simulink model "fwv_2020bn"  (R2020b)
settings: Solver=daessc  StartTime=0.0  StopTime=12  FixedStep=0.01  MaxStep=0.01  RelTol=1e-3  AbsTol=1e-3  EnableMultiTasking=on
model workspace: external: MATLAB File main.m (data not in the file)
values from neighbouring files (symbols this model uses):
  A_D = 1.5    [main.m]    (also in param.m; params.m)
  A_L = 1.8    [main.m]    (also in param.m; params.m)
  c_bar = S/R    (= 0.0357142857143)    [main.m]    (also in param.m = 0.0251327412287; params.m)
  C_D0 = 0.45    [main.m]    (also in param.m; params.m)
  m = 2    [rbf_pid.m]
  r00 = double(int(f,[0,1]))    [main.m]    (also in param.m = 1; params.m = 0.933333333333)
  r11 = double(int(x*f,[0,1]))    [main.m]    (also in param.m = double(int(curv(x)*(x+1/9),0,1)); params.m = 0.481185185185)
  r22 = double(int(x^2*f,[0,1]))    [main.m]    (also in param.m = double(int(curv(x)*(x+1/9)^2,0,1)); params.m = 0.304750617284)
  r33 = double(int(x^3*f,[0,1]))    [main.m]    (also in param.m = double(int(curv(x)*(x+1/9)^3,0,1)); params.m = 0.218568691358)
  r_cp = Rw*r33/r22    [main.m]    (also in param.m; params.m = 0.10758076225)
  rho = 1.205    [main.m]    (also in param.m; params.m)
  Rw = 0.15    [main.m]    (also in param.m = 0.075; params.m)
  z00 = double(int(f^2,[0,1]))    [main.m]    (also in param.m = double(int(curv(x)^2,0,1)); params.m = 1.00177777778)
  z11 = double(int(x*f^2,[0,1]))    [main.m]    (also in param.m = double(int(curv(x)^2*(x+1/9),0,1)); params.m = 0.484918518519)
  z22 = double(int(x^2*f^2,[0,1]))    [main.m]    (also in param.m = double(int(curv(x)^2*(x+1/9)^2,0,1)); params.m = 0.28785382716)
  zrd = double(int(f^4,[0,1]))    [main.m]    (also in param.m = double(int(curv(x)^4,0,1)); params.m = 1.29333866667)
undefined symbols (not defined in the file or in its folder): X, Y, Z
libraries: sm_lib x50, nesl_utility x45, pid_lib x5
(part 3 of 3)

== system fwv_2020bn/Controller/Subsystem/Outer PID ==
  In1 : Inport
  Demux : Demux  Outputs=3
  PID : Subsystem  mask{Kp=0.5, Ki=0.4, Kd=0.2, td=0}
  PID Controller1 : pid_lib/PID Controller  Controller=PID  Form=Parallel  TimeDomain=Continuous-time  UseExternalTs=off  SampleTime=-1  IntegratorMethod=Forward Euler  FilterMethod=Forward Euler  ControllerParametersSource=internal  P=0.3  I=0  D=0.3  UseFilter=on  N=25  TunerSelectOption=Transfer Function Based (PID Tuner App)  InitialConditionSource=internal  InitialConditionForIntegrator=0  InitialConditionForFilter=0  DifferentiatorICPrevScaledInput=0  ExternalReset=none  TrackingMode=off  Kt=1  LimitOutput=off  SatLimitsSource=internal  UpperSaturationLimit=inf  LowerSaturationLimit=-inf  LinearizeAsGain=on  AntiWindupMode=none  Kb=1  POutMin=[]  POutMax=[]  IOutMin=[]  IOutMax=[]  DOutMin=[]  DOutMax=[]  NOutMin=[]  NOutMax=[]  SumOutMin=[]  SumOutMax=[]  SaturationOutMin=[]  SaturationOutMax=[]  PParamMin=[]  PParamMax=[]  IParamMin=[]  IParamMax=[]  DParamMin=[]  DParamMax=[]  NParamMin=[]  NParamMax=[]  KbParamMin=[]  KbParamMax=[]  KtParamMin=[]  KtParamMax=[]  KbOutMin=[]  KbOutMax=[]  KtOutMin=[]  KtOutMax=[]  IntegratorOutMin=[]  IntegratorOutMax=[]  FilterOutMin=[]  FilterOutMax=[]  SumI1OutMin=[]  SumI1OutMax=[]  SumI2OutMin=[]  SumI2OutMax=[]  SumI3OutMin=[]  SumI3OutMax=[]  SumI4OutMin=[]  SumI4OutMax=[]  SumDOutMin=[]  SumDOutMax=[]  DifferentiatorOutMin=[]  DifferentiatorOutMax=[]  FilterDiffOutCoefMin=[]  FilterDiffOutCoefMax=[]  ReciprocalOutMin=[]  ReciprocalOutMax=[]  SumDenOutMin=[]  SumDenOutMax=[]  SumNumOutMin=[]  SumNumOutMax=[]  DivideOutMin=[]  DivideOutMax=[]  UdiffTsProdOutMin=[]  UdiffTsProdOutMax=[]  NTsProdOutMin=[]  NTsProdOutMax=[]  UintegralTsProdOutMin=[]  UintegralTsProdOutMax=[]  UngainTsProdOutMin=[]  UngainTsProdOutMax=[]  IntegratorContinuousStateAttributes=''  IntegratorStateMustResolveToSignalObject=off  IntegratorRTWStateStorageClass=Auto  FilterContinuousStateAttributes=''  FilterStateMustResolveToSignalObject=off  FilterRTWStateStorageClass=Auto  ParallelPVariant=InternalParameters  IdealPVariant=Disabled  IVariant=InternalParameters  DVariant=InternalParameters  IntegratorVariant=Continuous  SatVariant=Disabled  AWVariant=Passthrough  PCopyVariant=Disabled  TRVariant=Disabled  FdbkBlocksVariant=Forward  IdealPFdbkVariant=Disabled  SatFdbkVariant=Disabled  DerivativeFilterVariant=ContFilter  NVariant=InternalParameters  NCopyVariant=Disabled  FilterICVariant=InternalICsFilter  IntegratorICVariant=InternalICs  ExternalResetVariant=Disabled  TRSumVariant=Passthrough  SumFdbkVariant=Disabled  SumVariant=Sum_PID  TsampFilterVariant=InternalTs  TsampNgainVariant=Passthrough  TsampIntegralVariant=Passthrough  ExternalSaturationOutDataTypeStr=Inherit: Same as second input
  PID Controller2 : pid_lib/PID Controller  Controller=PID  Form=Parallel  TimeDomain=Continuous-time  UseExternalTs=off  SampleTime=-1  IntegratorMethod=Forward Euler  FilterMethod=Forward Euler  ControllerParametersSource=internal  P=0.3  I=0  D=0.3  UseFilter=on  N=25  TunerSelectOption=Transfer Function Based (PID Tuner App)  InitialConditionSource=internal  InitialConditionForIntegrator=0  InitialConditionForFilter=0  DifferentiatorICPrevScaledInput=0  ExternalReset=none  TrackingMode=off  Kt=1  LimitOutput=off  SatLimitsSource=internal  UpperSaturationLimit=inf  LowerSaturationLimit=-inf  LinearizeAsGain=on  AntiWindupMode=none  Kb=1  POutMin=[]  POutMax=[]  IOutMin=[]  IOutMax=[]  DOutMin=[]  DOutMax=[]  NOutMin=[]  NOutMax=[]  SumOutMin=[]  SumOutMax=[]  SaturationOutMin=[]  SaturationOutMax=[]  PParamMin=[]  PParamMax=[]  IParamMin=[]  IParamMax=[]  DParamMin=[]  DParamMax=[]  NParamMin=[]  NParamMax=[]  KbParamMin=[]  KbParamMax=[]  KtParamMin=[]  KtParamMax=[]  KbOutMin=[]  KbOutMax=[]  KtOutMin=[]  KtOutMax=[]  IntegratorOutMin=[]  IntegratorOutMax=[]  FilterOutMin=[]  FilterOutMax=[]  SumI1OutMin=[]  SumI1OutMax=[]  SumI2OutMin=[]  SumI2OutMax=[]  SumI3OutMin=[]  SumI3OutMax=[]  SumI4OutMin=[]  SumI4OutMax=[]  SumDOutMin=[]  SumDOutMax=[]  DifferentiatorOutMin=[]  DifferentiatorOutMax=[]  FilterDiffOutCoefMin=[]  FilterDiffOutCoefMax=[]  ReciprocalOutMin=[]  ReciprocalOutMax=[]  SumDenOutMin=[]  SumDenOutMax=[]  SumNumOutMin=[]  SumNumOutMax=[]  DivideOutMin=[]  DivideOutMax=[]  UdiffTsProdOutMin=[]  UdiffTsProdOutMax=[]  NTsProdOutMin=[]  NTsProdOutMax=[]  UintegralTsProdOutMin=[]  UintegralTsProdOutMax=[]  UngainTsProdOutMin=[]  UngainTsProdOutMax=[]  IntegratorContinuousStateAttributes=''  IntegratorStateMustResolveToSignalObject=off  IntegratorRTWStateStorageClass=Auto  FilterContinuousStateAttributes=''  FilterStateMustResolveToSignalObject=off  FilterRTWStateStorageClass=Auto  ParallelPVariant=InternalParameters  IdealPVariant=Disabled  IVariant=InternalParameters  DVariant=InternalParameters  IntegratorVariant=Continuous  SatVariant=Disabled  AWVariant=Passthrough  PCopyVariant=Disabled  TRVariant=Disabled  FdbkBlocksVariant=Forward  IdealPFdbkVariant=Disabled  SatFdbkVariant=Disabled  DerivativeFilterVariant=ContFilter  NVariant=InternalParameters  NCopyVariant=Disabled  FilterICVariant=InternalICsFilter  IntegratorICVariant=InternalICs  ExternalResetVariant=Disabled  TRSumVariant=Passthrough  SumFdbkVariant=Disabled  SumVariant=Sum_PID  TsampFilterVariant=InternalTs  TsampNgainVariant=Passthrough  TsampIntegralVariant=Passthrough  ExternalSaturationOutDataTypeStr=Inherit: Same as second input
  mux : Outport
  muy : Outport  Port=2
  muz : Outport  Port=3
  wires:
  Demux/1 -> PID Controller2/1
  Demux/2 -> PID Controller1/1
  PID Controller2/1 -> mux/1
  PID Controller1/1 -> muy/1
  PID/1(Out1) -> muz/1
  Demux/3 -> PID/1(In1)
  In1/1 -> Demux/1

== system fwv_2020bn/FWV/LEFT WING/Subsystem1 ==
  Gain : Gain  Gain=-1
  LWing-root in world : sm_lib/Frames and Transforms/Transform Sensor  MeasurementFrame=NonRotatingFollower  SenseAngle=off  SenseAxis=off  SenseAngle1=off  SenseAngle2=off  SenseAngle3=off  SenseQ=off  SenseR=off  SenseOmegaX=on  SenseOmegaY=on  SenseOmegaZ=off  SenseOmega1=off  SenseOmega2=off  SenseOmega3=off  SenseQDot=off  SenseRDot=off  SenseAlphaX=off  SenseAlphaY=off  SenseAlphaZ=off  SenseAlpha1=off  SenseAlpha2=off  SenseAlpha3=off  SenseQDDot=off  SenseRDDot=off  SenseX=off  SenseY=off  SenseZ=off  SenseRad=off  SenseAzim=off  SenseDist=off  SenseInc=off  SenseXDot=on  SenseYDot=on  SenseZDot=off  SenseRadDot=off  SenseAzimDot=off  SenseDistDot=off  SenseIncDot=off  SenseXDDot=off  SenseYDDot=off  SenseZDDot=off  SenseRadDDot=off  SenseAzimDDot=off  SenseDistDDot=off  SenseIncDDot=off
  Mux : Mux
  PS-Simulink Converter{,1..3} (4 alike) : nesl_utility/PS-Simulink Converter  PhysicalDomain=network_engine_domain  SubClassName=ps_output  LeftPortType=input  RightPortType=output  PseudoPeriodic=off  Frequencies=[]  Unit=inherit  AffineConversion=off
      settings: SourceProductBaseCode=PW,SS
  W : PMIOPort  Side=Left
  WT : PMIOPort  Port=2  Side=Left
  le0 : Outport
  wires:
  Mux/1 -> le0/1
  Gain/1 -> Mux/2
  PS-Simulink Converter1/1 -> Mux/3
  PS-Simulink Converter3/1 -> Gain/1
  PS-Simulink Converter2/1 -> Mux/1
  PS-Simulink Converter/1 -> Mux/4
  connections:
  W/RConn1 -- LWing-root in world/LConn1
  WT/RConn1 -- LWing-root in world/RConn1
  LWing-root in world/RConn2 -- PS-Simulink Converter/LConn1
  LWing-root in world/RConn3 -- PS-Simulink Converter1/LConn1
  LWing-root in world/RConn4 -- PS-Simulink Converter2/LConn1
  LWing-root in world/RConn5 -- PS-Simulink Converter3/LConn1

== system fwv_2020bn/FWV/RIGHT WING/Subsystem1 ==
  Gain : Gain  Gain=-1
  LWing-root in world : sm_lib/Frames and Transforms/Transform Sensor  MeasurementFrame=NonRotatingFollower  SenseAngle=off  SenseAxis=off  SenseAngle1=off  SenseAngle2=off  SenseAngle3=off  SenseQ=off  SenseR=off  SenseOmegaX=on  SenseOmegaY=on  SenseOmegaZ=off  SenseOmega1=off  SenseOmega2=off  SenseOmega3=off  SenseQDot=off  SenseRDot=off  SenseAlphaX=off  SenseAlphaY=off  SenseAlphaZ=off  SenseAlpha1=off  SenseAlpha2=off  SenseAlpha3=off  SenseQDDot=off  SenseRDDot=off  SenseX=off  SenseY=off  SenseZ=off  SenseRad=off  SenseAzim=off  SenseDist=off  SenseInc=off  SenseXDot=on  SenseYDot=on  SenseZDot=off  SenseRadDot=off  SenseAzimDot=off  SenseDistDot=off  SenseIncDot=off  SenseXDDot=off  SenseYDDot=off  SenseZDDot=off  SenseRadDDot=off  SenseAzimDDot=off  SenseDistDDot=off  SenseIncDDot=off
  Mux : Mux
  PS-Simulink Converter{,1..3} (4 alike) : nesl_utility/PS-Simulink Converter  PhysicalDomain=network_engine_domain  SubClassName=ps_output  LeftPortType=input  RightPortType=output  PseudoPeriodic=off  Frequencies=[]  Unit=inherit  AffineConversion=off
      settings: SourceProductBaseCode=PW,SS
  W : PMIOPort  Side=Left
  WT : PMIOPort  Port=2  Side=Left
  le0 : Outport
  wires:
  Mux/1 -> le0/1
  Gain/1 -> Mux/2
  PS-Simulink Converter1/1 -> Mux/3
  PS-Simulink Converter3/1 -> Gain/1
  PS-Simulink Converter2/1 -> Mux/1
  PS-Simulink Converter/1 -> Mux/4
  connections:
  W/RConn1 -- LWing-root in world/LConn1
  WT/RConn1 -- LWing-root in world/RConn1
  LWing-root in world/RConn2 -- PS-Simulink Converter/LConn1
  LWing-root in world/RConn3 -- PS-Simulink Converter1/LConn1
  LWing-root in world/RConn4 -- PS-Simulink Converter2/LConn1
  LWing-root in world/RConn5 -- PS-Simulink Converter3/LConn1

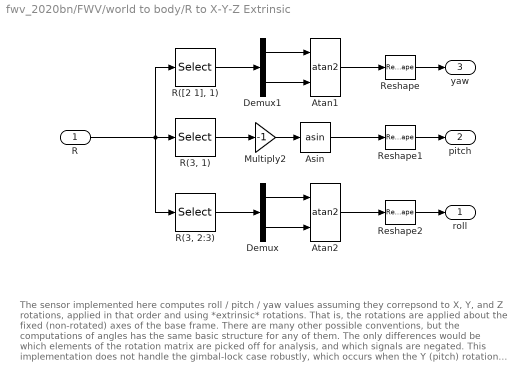
== system fwv_2020bn/FWV/world to body/R to X-Y-Z Extrinsic ==
  note: The sensor implemented here computes roll / pitch / yaw values assuming they correpsond to X, Y, and Z rotations, applied in that order and using  *extrinsic* rotations.  That is, the rotations are applied about the fixed (non-rotated) axes of the base frame.   There are many other possible conventions, but the computations of angles has the same basic structure for any of them.  The only differences would be which elements of the rotation matrix are picked off for analysis, and which signals are negated.
      |
      | This implementation does not handle the gimbal-lock case robustly, which occurs when the Y (pitch) rotation is +/-90 degrees.  Handling this case requires a more complex computation,
      | but it can be done with a few more trig blocks and selectors.
  R : Inport
  Asin : Trigonometry  Operator=asin
  Atan1 : Trigonometry  Operator=atan2
  Atan2 : Trigonometry  Operator=atan2
  Demux : Demux  Outputs=2
  Demux1 : Demux  Outputs=2
  Multiply2 : Gain  Gain=-1
  "R(3, 1)" : Selector  NumberOfDimensions=2  InputPortWidth=3  IndexOptions=Index vector (dialog),Index vector (dialog)  Indices=3,1  OutputSizes=1,1
  "R(3, 2:3)" : Selector  NumberOfDimensions=2  InputPortWidth=3  IndexOptions=Index vector (dialog),Index vector (dialog)  Indices=3,[2 3]  OutputSizes=1,1
  "R([2 1], 1)" : Selector  NumberOfDimensions=2  InputPortWidth=3  IndexOptions=Index vector (dialog),Index vector (dialog)  Indices=[2 1],1  OutputSizes=1,1
  Reshape : Reshape
  Reshape1 : Reshape
  Reshape2 : Reshape  OutputDimensionality=Customize  OutputDimensions=1
  roll : Outport  VectorParamsAs1DForOutWhenUnconnected=off
  pitch : Outport  Port=2  VectorParamsAs1DForOutWhenUnconnected=off
  yaw : Outport  Port=3  VectorParamsAs1DForOutWhenUnconnected=off
  wires:
  Demux/1 -> Atan2/1
  Demux1/2 -> Atan1/2
  Demux/2 -> Atan2/2
  Atan2/1 -> Reshape2/1
  "R(3, 1)"/1 -> Multiply2/1
  Asin/1 -> Reshape1/1
  R/1 -> "R(3, 1)"/1, "R(3, 2:3)"/1, "R([2 1], 1)"/1
  Demux1/1 -> Atan1/1
  "R([2 1], 1)"/1 -> Demux1/1
  Multiply2/1 -> Asin/1
  "R(3, 2:3)"/1 -> Demux/1
  Atan1/1 -> Reshape/1
  Reshape/1 -> yaw/1
  Reshape1/1 -> pitch/1
  Reshape2/1 -> roll/1

== system fwv_2020bn/Controller/Subsystem/Outer PID/PID ==
  In1 : Inport
  Constant : Constant  Value=Kp
  Constant1 : Constant  Value=Ki
  Constant2 : Constant  Value=Kd
  Derivative : Derivative  CoefficientInTFapproximation=0.2
  Dot Product : DotProduct  InputSameDT=on  OutDataTypeStr=Inherit: Inherit via internal rule
  Integrator Limited : Integrator  LimitOutput=on  UpperSaturationLimit=15  LowerSaturationLimit=-15
  Mux : Mux  Inputs=3
  Mux1 : Mux  Inputs=3
  Out1 : Outport
  wires:
  In1/1 -> Derivative/1, Mux/1, Integrator Limited/1
  Dot Product/1 -> Out1/1
  Integrator Limited/1 -> Mux/2
  Derivative/1 -> Mux/3
  Mux/1 -> Dot Product/2
  Constant1/1 -> Mux1/2
  Constant/1 -> Mux1/1
  Constant2/1 -> Mux1/3
  Mux1/1 -> Dot Product/1

== matlab function fwv_2020bn/FWV/RIGHT WING/right aero force and moment ==
  data: le0 input; F_N output; alpha input; M_rd output; d_cp output; rot_dot input; A_L parameter; A_D parameter; C_D0 parameter; rho parameter; c_bar parameter; Rw parameter; r22 parameter; r11 parameter; r00 parameter; z22 parameter; z11 parameter; z00 parameter; zrd parameter
function [F_N,M_rd,d_cp]= fcn(le0, alpha, rot_dot, A_L, A_D, C_D0, rho, c_bar, Rw, r22, r11, r00, z22, z11, z00, zrd)
a2=le0(3)^2+le0(4)^2;
a1=-2*(le0(1)*le0(3)+le0(2)*le0(4));
a0=le0(1)^2+le0(2)^2;
C_L=A_L*sin(2*alpha);
C_D=C_D0+A_D*(1-cos(2*alpha));
C_N=C_L*cos(alpha)+C_D*sin(alpha);
C_A=C_L*sin(alpha)-C_D*cos(alpha);
F_N = -0.5*rho*C_N*c_bar*(a2*Rw^3*r22+a1*Rw^2*r11+a0*Rw*r00);
d_cp_=0.82/pi*(mod(abs(alpha),pi))+0.05;
M_ae=-0.5*rho*C_N*c_bar^2*d_cp_*(a2*Rw^3*z22+a1*Rw^2*z11+a0*Rw*z00);
if F_N==0
    d_cp=-0.51*c_bar;
else
    d_cp=-M_ae/F_N;
end
M_rd=-0.125*rho*5*rot_dot*abs(rot_dot)*Rw*c_bar^4*zrd;

== matlab function fwv_2020bn/FWV/Acuator/ left flap ==
  data: t input; y output; amp input; sig input; freq input; bias input
function y = flap(t,amp,sig,freq,bias)
tn = mod(freq*t,1);
if tn<sig
    y = amp*cos(2*pi*tn/(2*sig))+bias;
else
    y = amp*cos(2*pi*(1-tn)/(2-2*sig))+bias;
end
if abs(y)>pi/2
    y = sign(y)*pi/2;
end

== matlab function fwv_2020bn/FWV/Acuator/ right flap ==
  data: t input; y output; amp input; sig input; freq input; bias input
function y = flap(t,amp,sig,freq,bias)
sig=1-sig;
tn = mod(freq*t,1);
if tn<sig
    y = amp*cos(2*pi*tn/(2*sig))+bias;
else
    y = amp*cos(2*pi*(1-tn)/(2-2*sig))+bias;
end
if abs(y)>pi/2
    y = sign(y)*pi/2;
end

== matlab function fwv_2020bn/Controller/Subsystem/inner-outer convertion ==
  data: mux input; etad output; muy input; muz input; psid input; ufz output
function [etad,ufz] = fcn(mux,muy,muz,psid)

m = 0.024;
ufd =  m * sqrt(mux^2+muy^2+(muz)^2);
ufz = m * (muz+9.806);
if muz==0
    etad = [0,0,0];
else
phid = asin(m*(mux*sin(psid)-muy*cos(psid))/ufd);
thetad = atan((mux*cos(psid)+muy*sin(psid))/muz);
etad = [phid,thetad,psid];
end

== matlab function fwv_2020bn/FWV/LEFT WING/AoA ==
  data: le0 input; alpha output; rot input; Rw parameter; r33 parameter; r22 parameter
function alpha = fcn(le0, rot, Rw, r33, r22)
rcp = Rw*r33/r22;
vi = le0(1)+le0(3)*rcp;
vo = le0(2)+le0(4)*rcp;
dir_v = atan2(vo,vi);
if vi~=0
    alpha = -rot + sign(vi)*pi/2 - atan(vo/vi);
else
    alpha = 0;
end

== matlab function fwv_2020bn/FWV/LEFT WING/left aero force and moment ==
  data: le0 input; F_N output; alpha input; M_rd output; d_cp output; rot_dot input; A_L parameter; A_D parameter; C_D0 parameter; rho parameter; c_bar parameter; Rw parameter; r22 parameter; r11 parameter; r00 parameter; z22 parameter; z11 parameter; z00 parameter; zrd parameter
function [F_N, M_rd, d_cp] = fcn(le0, alpha, rot_dot, A_L, A_D, C_D0, rho, c_bar, Rw, r22, r11, r00, z22, z11, z00, zrd)
a2=le0(3)^2+le0(4)^2;
a1=2*(le0(1)*le0(3)+le0(2)*le0(4));
a0=le0(1)^2+le0(2)^2;
C_L=A_L*sin(2*alpha);
C_D=C_D0+A_D*(1-cos(2*alpha));
C_N=C_L*cos(alpha)+C_D*sin(alpha);
C_A=C_L*sin(alpha)-C_D*cos(alpha);
F_N = -0.5*rho*C_N*c_bar*(a2*Rw^3*r22+a1*Rw^2*r11+a0*Rw*r00);
d_cp_=0.82/pi*(mod(abs(alpha),pi))+0.05;
M_ae=-0.5*rho*C_N*c_bar^2*d_cp_*(a2*Rw^3*z22+a1*Rw^2*z11+a0*Rw*z00);
if F_N==0
    d_cp=-0.51*c_bar;
else
    d_cp = -M_ae/F_N;
end
M_rd=-0.125*rho*5*rot_dot*abs(rot_dot)*Rw*c_bar^4*zrd;

== matlab function fwv_2020bn/FWV/RIGHT WING/AoA1 ==
  data: le0 input; alpha output; rot input; Rw parameter; r33 parameter; r22 parameter
function alpha = fcn(le0, rot, Rw, r33, r22)
rcp = -Rw*r33/r22;
vi = le0(1)+le0(3)*rcp;
vo = le0(2)+le0(4)*rcp;
if vi~=0
    alpha = -rot + sign(vi)*pi/2 - atan(vo/vi);
else
    alpha = 0;
end
